simulink model "c28x_i2c_eeprom_interrupt"  (R2021b)
settings: Solver=FixedStepDiscrete  StartTime=0.0  StopTime=Inf  FixedStep=0.2  RelTol=1e-3  EnableMultiTasking=on
libraries: simulink x9, c280xlib x3, demo_controls x1, c2000lib x1, idelinklib_common x1
settings Model: SimulationMode=external  ExtModeTrigDuration=8  Creator=The MathWorks, Inc.  LastModifiedBy=The MathWorks, Inc.
settings SolverCC: AlgebraicLoopSolver=TrustRegion
settings DataIOCC: LimitDataPoints=on  SaveFormat=Array  SaveOutput=off  SaveTime=off  ReturnWorkspaceOutputs=off
settings OptimizationCC: DefaultUnderspecifiedDataType=single  ExpressionDepthLimit=2147483647  InitFltsAndDblsToZero=on  LifeSpan=inf  MaxStackSize=512  EfficientTunableParamExpr=on
settings DebuggingCC: ReadBeforeWriteMsg=DisableAll  UnderspecifiedInitializationDetection=Classic  MergeDetectMultiDrivingBlocksExec=none  SolverPrmCheckMsg=warning  InheritedTsInSrcMsg=none  MultiTaskDSMMsg=none  FcnCallInpInsideContextMsg=warning  AllowSymbolicDim=off  StateNameClashWarn=warning  SFUnexpectedBacktrackingDiag=warning  SFNoUnconditionalDefaultTransitionDiag=warning  SFExecutionAtInitializationDiag=none  SFMachineParentedDataDiag=warning  ArithmeticOperatorsInVariantConditions=warning
settings HardwareCC: ProdBitPerChar=16  ProdBitPerInt=16  ProdBitPerPointer=32  ProdBitPerSizeT=32  ProdBitPerPtrDiffT=32  ProdLargestAtomicInteger=Integer  ProdLargestAtomicFloat=None  ProdWordSize=16  ProdLongLongMode=on  ProdHWDeviceType=Texas Instruments->C2000  TargetBitPerChar=16  TargetBitPerInt=16  TargetLargestAtomicInteger=Integer  TargetIntDivRoundTo=Zero  TargetEndianess=LittleEndian  TargetWordSize=16  TargetHWDeviceType=Texas Instruments->C2000  ProdEqTarget=off
settings ModelReferenceCC: PropagateSignalLabelsOutOfModel=off
settings SFSimCC: SimUseLocalCustomCode=off  SimParseCustomCode=off  CustomCodeUndefinedFunction=UseInterfaceOnly
settings RTWCC: Description=Embedded Coder  SystemTargetFile=ert.tlc  HardwareBoard=TI Delfino F2833x  TemplateMakefile=ert_default_tmf  RTWUseLocalCustomCode=off  Toolchain=Texas Instruments Code Composer Studio (C2000)  BuildConfiguration=Specify
settings CodeAppCC: IgnoreCustomStorageClasses=off  CustomSymbolStrType=$N$R$M  StateflowObjectComments=on  InternalIdentifier=Classic
settings ERTTargetCC: CodeReplacementLibrary=TI C28x  MultiwordLength=2048  ParMdlRefBuildCompliant=off  CPPClassGenCompliant=off  ExtModeTransport=4  ExtModeStaticAlloc=on  ExtModeStaticAllocSize=2048  ExtModeMexFile=ext_xcp  ExtModeIntrfLevel=Level2 - Open  ConvertIfToSwitch=off  SuppressUnreachableDefaultCases=off
settings ConfigComp: CovMetricSettings=dw  CovSaveCumulativeToWorkspaceVar=on  CovSaveSingleToWorkspaceVar=on  CovExternalEMLEnable=off  CovSFcnEnable=off

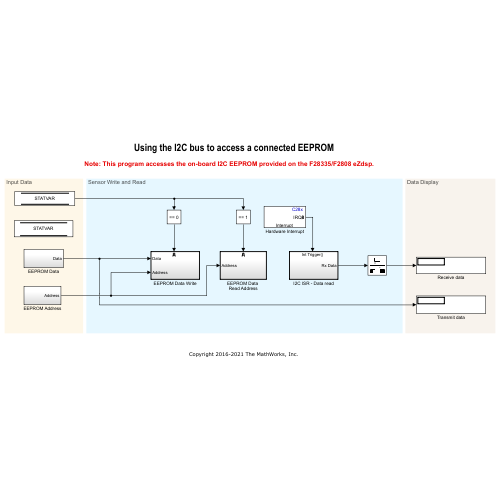
[thumbnail: Simulink's stored preview of the top-level diagram]
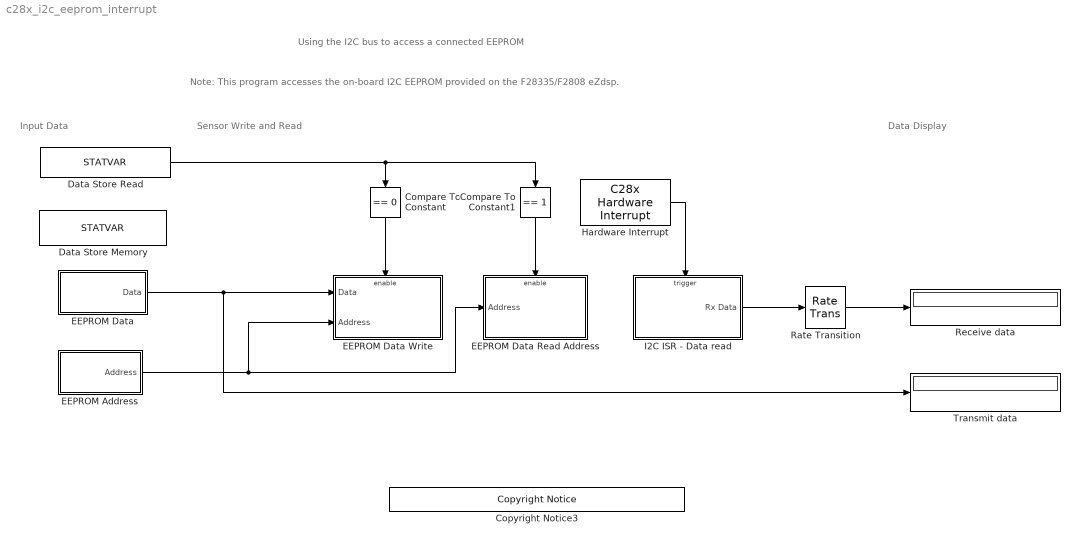
== system c28x_i2c_eeprom_interrupt ==
  note: Using the I2C bus to access a connected EEPROM
  note: Note: This program accesses the on-board I2C EEPROM provided on the F28335/F2808 eZdsp.
  note: Input Data
  note: Sensor Write and Read
  note: Data Display
  Compare To Constant : simulink/Logic and Bit Operations/Compare To Constant  relop===  const=0  OutDataTypeStr=boolean  ZeroCross=off
  Compare To Constant1 : simulink/Logic and Bit Operations/Compare To Constant  relop===  const=1  OutDataTypeStr=boolean  ZeroCross=off
  Copyright Notice3 : demo_controls/Copyright Notice  year=2016  prod=tic2000
      settings: SourceProductBaseCode=ME
  Data Store Memory : DataStoreMemory  DataStoreName=STATVAR  ReadBeforeWriteMsg=warning  WriteAfterWriteMsg=warning  WriteAfterReadMsg=warning  ShowAdditionalParam=off  OutDataTypeStr=uint16
  Data Store Read : DataStoreRead  DataStoreName=STATVAR  IndexOptions=Index vector (dialog)  Indices=1  OutputSizes=1
  EEPROM Address : Subsystem
  EEPROM Data : Subsystem
  EEPROM Data Read Address : Subsystem
  EEPROM Data Write : Subsystem
  Hardware Interrupt : c2000lib/Scheduling/C28x Hardware Interrupt  irqnumbers=8  pienumbers=1  irqpriorities=30  irqpreempts=1  showinput=off  dspchiptype=C280X
      settings: SourceProductBaseCode=TIC2000
  I2C ISR - Data read : Subsystem
  Rate Transition : RateTransition  Deterministic=off
  Receive data : Display
  Transmit data : Display
  wires:
  I2C ISR - Data read/1(Rx Data) -> Rate Transition/1
  EEPROM Address/1(Address) -> EEPROM Data Write/2(Address), EEPROM Data Read Address/1(Address)
  EEPROM Data/1(Data) -> EEPROM Data Write/1(Data), Transmit data/1
  Hardware Interrupt/1 -> I2C ISR - Data read/Trigger
  Compare To Constant/1 -> EEPROM Data Write/Enable
  Data Store Read/1 -> Compare To Constant1/1, Compare To Constant/1
  Compare To Constant1/1 -> EEPROM Data Read Address/Enable
  Rate Transition/1 -> Receive data/1

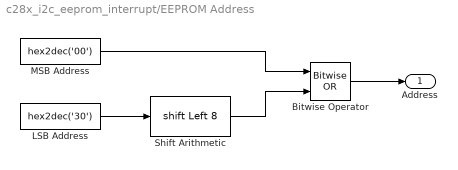
== system c28x_i2c_eeprom_interrupt/EEPROM Address ==
  Bitwise Operator : simulink/Logic and Bit Operations/Bitwise Operator  logicop=OR  UseBitMask=off  NumInputPorts=2  BitMask=bin2dec('11011001')  BitMaskRealWorld=Stored Integer
  LSB Address : Constant  Value=hex2dec('30')  OutDataTypeStr=uint16  SampleTime=-1
  MSB Address : Constant  Value=hex2dec('00')  OutDataTypeStr=uint16  SampleTime=-1
  Shift Arithmetic : ArithShift  BitShiftNumber=8  BitShiftDirection=Left
  Address : Outport  VectorParamsAs1DForOutWhenUnconnected=off
  wires:
  LSB Address/1 -> Shift Arithmetic/1
  MSB Address/1 -> Bitwise Operator/1
  Shift Arithmetic/1 -> Bitwise Operator/2
  Bitwise Operator/1 -> Address/1

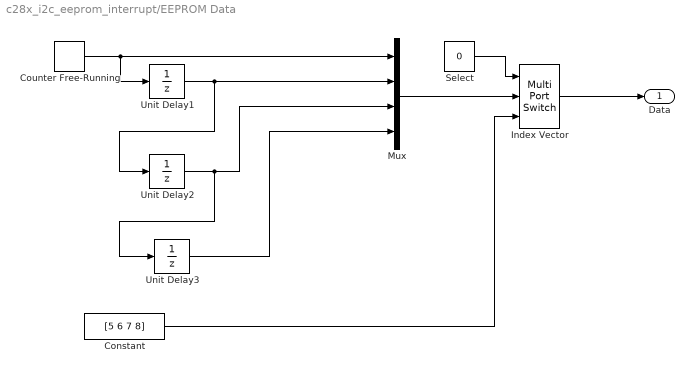
== system c28x_i2c_eeprom_interrupt/EEPROM Data ==
  Constant : Constant  Value=[5 6 7 8]  OutDataTypeStr=uint8  SampleTime=-1
  Counter Free-Running : simulink/Sources/Counter Free-Running  NumBits=8  tsamp=-1
  Index Vector : MultiPortSwitch  DataPortOrder=Zero-based contiguous  Inputs=2  zeroidx=on  OutDataTypeStr=uint16
  Mux : Mux
  Select : Constant  Value=0  SampleTime=-1
  Unit Delay1 : UnitDelay  SampleTime=-1  HasFrameUpgradeWarning=on
  Unit Delay2 : UnitDelay  SampleTime=-1  HasFrameUpgradeWarning=on
  Unit Delay3 : UnitDelay  SampleTime=-1  HasFrameUpgradeWarning=on
  Data : Outport  VectorParamsAs1DForOutWhenUnconnected=off
  wires:
  Unit Delay1/1 -> Unit Delay2/1, Mux/2
  Unit Delay2/1 -> Mux/3, Unit Delay3/1
  Unit Delay3/1 -> Mux/4
  Mux/1 -> Index Vector/2
  Constant/1 -> Index Vector/3
  Index Vector/1 -> Data/1
  Select/1 -> Index Vector/1
  Counter Free-Running/1 -> Unit Delay1/1, Mux/1

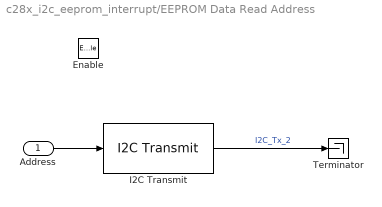
== system c28x_i2c_eeprom_interrupt/EEPROM Data Read Address ==
  Address : Inport
  Enable : EnablePort  PropagateVarSize=During execution
  I2C Transmit : c280xlib/I2C Transmit  Priority=1  selectModule=I2C_A  addrFormat=7-Bit addressing  saSource=Specify via dialog  SAR=hex2dec('50')  bitCount=8  STP=off  RM=off  STR=on
      settings: SourceProductBaseCode=TIC2000
  Terminator : Terminator
  wires:
  I2C Transmit/1 -> Terminator/1  "I2C_Tx_2"
  Address/1 -> I2C Transmit/1

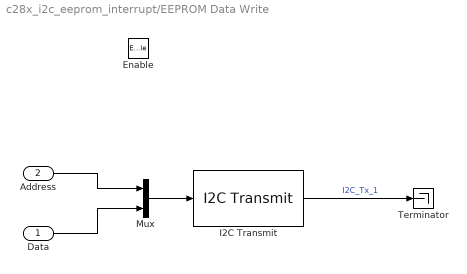
== system c28x_i2c_eeprom_interrupt/EEPROM Data Write ==
  Data : Inport
  Address : Inport  Port=2
  Enable : EnablePort  PropagateVarSize=During execution
  I2C Transmit : c280xlib/I2C Transmit  Priority=2  selectModule=I2C_A  addrFormat=7-Bit addressing  saSource=Specify via dialog  SAR=hex2dec('50')  bitCount=8  STP=on  RM=off  STR=on
      settings: SourceProductBaseCode=TIC2000
  Mux : Mux  Inputs=2
  Terminator : Terminator
  wires:
  I2C Transmit/1 -> Terminator/1  "I2C_Tx_1"
  Mux/1 -> I2C Transmit/1
  Address/1 -> Mux/1
  Data/1 -> Mux/2

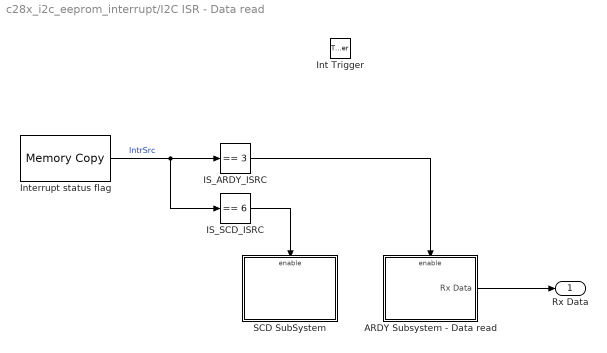
== system c28x_i2c_eeprom_interrupt/I2C ISR - Data read ==
  Int Trigger : TriggerPort  TriggerType=function-call  VariantControl=Variant
  ARDY Subsystem - Data read : Subsystem
  IS_ARDY_ISRC : simulink/Logic and Bit Operations/Compare To Constant  relop===  const=3  OutDataTypeStr=boolean  ZeroCross=off
  IS_SCD_ISRC : simulink/Logic and Bit Operations/Compare To Constant  relop===  const=6  OutDataTypeStr=boolean  ZeroCross=off
  Interrupt status flag : idelinklib_common/Memory Copy  copyFrom=Specified source code symbol  copyFromAddressSource=Specify via dialog  copyFromAddress=hex2dec('00001000')  copyFromSrcCode=&I2caRegs.I2CISRC.all  dataTypeFrom=uint16  dataDimensionFrom=1  useOffsetFrom=off  offsetFromSrc=Specify via dialog  offsetFrom=1  strideFrom=1  copyTo=Output port  copyToAddressSource=Specify via dialog  copyToAddress=hex2dec('00002000')  copyToSrcCode=myVariableDst  dataTypeTo=uint16  useOffsetTo=off  offsetToSrc=Specify via dialog  offsetTo=1  strideTo=1  sampleTime=-1  useInitValue=off  initValueSrc=Specify constant value  initValue=1  initValueSrcCode=myInitValueVariable  useAsMask=off  maskOperator=bitwise AND  useTermValue=off  termValue=1  isRealtimeEnabled=off  emitCCBeforeWrite=off  CCBeforeWrite=/* Custom Code Before Write*/  emitCCAfterWrite=off  CCAfterWrite=/* Custom Code After Write*/  useDMACopy=off  enableBlockingMode=off
      settings: SourceProductBaseCode=ME
  SCD SubSystem : Subsystem
  Rx Data : Outport  VectorParamsAs1DForOutWhenUnconnected=off
  wires:
  Interrupt status flag/1 -> IS_SCD_ISRC/1, IS_ARDY_ISRC/1  "IntrSrc"
  IS_ARDY_ISRC/1 -> ARDY Subsystem - Data read/Enable
  IS_SCD_ISRC/1 -> SCD SubSystem/Enable
  ARDY Subsystem - Data read/1(Rx Data) -> Rx Data/1

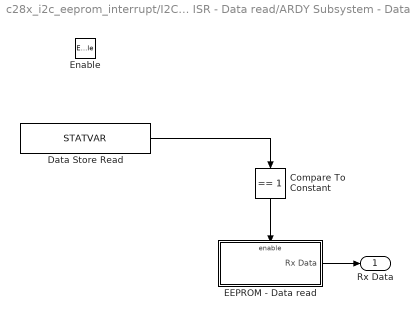
== system c28x_i2c_eeprom_interrupt/I2C ISR - Data read/ARDY Subsystem - Data read ==
  Enable : EnablePort  PropagateVarSize=During execution
  Compare To Constant : simulink/Logic and Bit Operations/Compare To Constant  relop===  const=1  OutDataTypeStr=boolean  ZeroCross=off
  Data Store Read : DataStoreRead  DataStoreName=STATVAR  IndexOptions=Index vector (dialog)  Indices=1  OutputSizes=1
  EEPROM - Data read : Subsystem
  Rx Data : Outport  VectorParamsAs1DForOutWhenUnconnected=off
  wires:
  Data Store Read/1 -> Compare To Constant/1
  Compare To Constant/1 -> EEPROM - Data read/Enable
  EEPROM - Data read/1(Rx Data) -> Rx Data/1

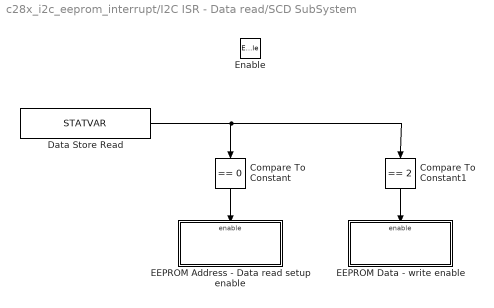
== system c28x_i2c_eeprom_interrupt/I2C ISR - Data read/SCD SubSystem ==
  Enable : EnablePort  PropagateVarSize=During execution
  Compare To Constant : simulink/Logic and Bit Operations/Compare To Constant  relop===  const=0  OutDataTypeStr=boolean  ZeroCross=off
  Compare To Constant1 : simulink/Logic and Bit Operations/Compare To Constant  relop===  const=2  OutDataTypeStr=boolean  ZeroCross=off
  Data Store Read : DataStoreRead  DataStoreName=STATVAR  IndexOptions=Index vector (dialog)  Indices=1  OutputSizes=1
  EEPROM Address - Data read setup enable : Subsystem
  EEPROM Data - write enable : Subsystem
  wires:
  Data Store Read/1 -> Compare To Constant1/1, Compare To Constant/1
  Compare To Constant/1 -> EEPROM Address - Data read setup enable/Enable
  Compare To Constant1/1 -> EEPROM Data - write enable/Enable

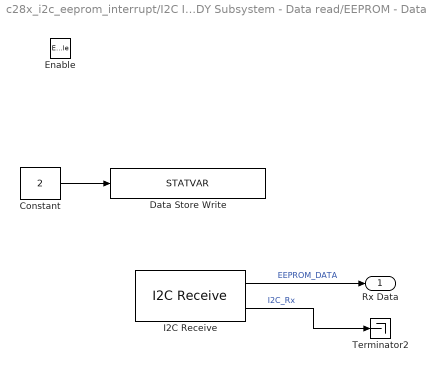
== system c28x_i2c_eeprom_interrupt/I2C ISR - Data read/ARDY Subsystem - Data read/EEPROM - Data read ==
  Enable : EnablePort  PropagateVarSize=During execution
  Constant : Constant  Value=2  OutDataTypeStr=uint16  SampleTime=-1
  Data Store Write : DataStoreWrite  DataStoreName=STATVAR  IndexOptions=Index vector (dialog)  Indices=1  OutputSizes=1
  I2C Receive : c280xlib/I2C Receive  selectModule=I2C_A  addrFormat=7-Bit addressing  saSource=Specify via dialog  SAR=hex2dec('50')  bitCount=8  dataLength=4  initValue=0  NACK=off  STP=on  STR=on  sampleTime=Inf  dataType=uint16
      settings: SourceProductBaseCode=TIC2000
  Terminator2 : Terminator
  Rx Data : Outport  VectorParamsAs1DForOutWhenUnconnected=off
  wires:
  Constant/1 -> Data Store Write/1
  I2C Receive/1 -> Rx Data/1  "EEPROM_DATA"
  I2C Receive/2 -> Terminator2/1  "I2C_Rx"

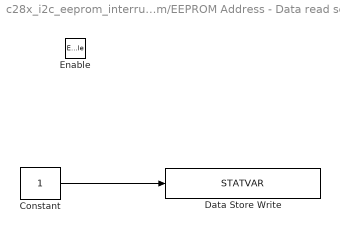
== system c28x_i2c_eeprom_interrupt/I2C ISR - Data read/SCD SubSystem/EEPROM Address - Data read setup enable ==
  Enable : EnablePort  PropagateVarSize=During execution
  Constant : Constant  OutDataTypeStr=uint16  SampleTime=-1
  Data Store Write : DataStoreWrite  DataStoreName=STATVAR  IndexOptions=Index vector (dialog)  Indices=1  OutputSizes=1
  wires:
  Constant/1 -> Data Store Write/1

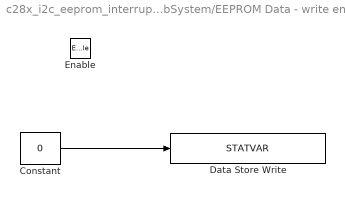
== system c28x_i2c_eeprom_interrupt/I2C ISR - Data read/SCD SubSystem/EEPROM Data - write enable ==
  Enable : EnablePort  PropagateVarSize=During execution
  Constant : Constant  Value=0  OutDataTypeStr=uint16  SampleTime=-1
  Data Store Write : DataStoreWrite  DataStoreName=STATVAR  IndexOptions=Index vector (dialog)  Indices=1  OutputSizes=1
  wires:
  Constant/1 -> Data Store Write/1
